simulink model "chap3_2"  (Simulink 5.0)
settings: Solver=ode5  StartTime=0.0  StopTime=500*T  FixedStep=T  RelTol=1e-3
PreLoadFcn:
  | T=0.001; Kp=0.6; Ki=0.03; Kd=0.01;

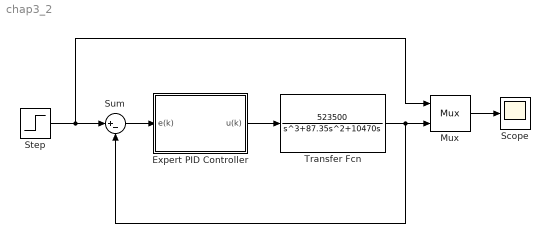
== system chap3_2 ==
  Expert PID Controller : Subsystem  mask{kp=Kp, ki=Ki, kd=Kd, T=0.001, MTab=[0.8,0.45; 0.4,0.4; 0.2,0.12; 0.01 0.1], U_m=10}
      mask prompts: kp "Proportional Kp"; ki "Integral Ki"; kd "Derivative Kd"; T "Sampling period T"; MTab "Mapping Table"; U_m "Actuator Limit U_m"
      mask Display: disp('Expert PID\n Controller')
  Mux : Mux  Inputs=2
  Scope : Scope
      settings: TimeRange=0.5  YMin=-0.0669643  YMax=1.10225  SaveName=yy  DataFormat=Array
  Step : Step  Time=0  SampleTime=0
  Sum : Sum  Inputs=|+-  SaturateOnIntegerOverflow=on  InputSameDT=on
  Transfer Fcn : TransferFcn  Numerator=[523500]  Denominator=[1 87.35 10470 0]
  wires:
  Transfer Fcn/1 -> Sum/2, Mux/2
  Step/1 -> Sum/1, Mux/1
  Expert PID Controller/1(u(k)) -> Transfer Fcn/1
  Sum/1 -> Expert PID Controller/1(e(k))
  Mux/1 -> Scope/1

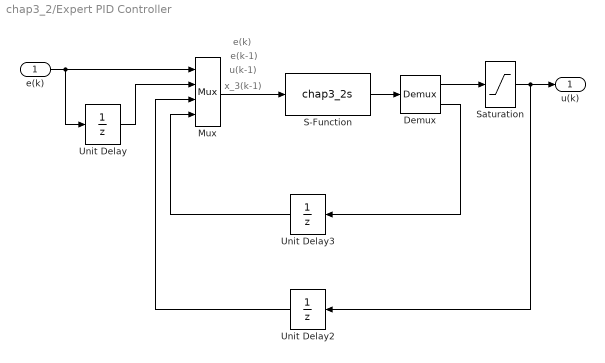
== system chap3_2/Expert PID Controller ==
  note: e(k)
  note: e(k-1)
  note: u(k-1)
  note: x_3(k-1)
  e(k) : Inport
  Demux : Demux  Outputs=2
  Mux : Mux
  S-Function : S-Function  FunctionName=chap3_2s  Parameters=T,Kp,Ki,Kd,MTab
  Saturation : Saturate  UpperLimit=U_m  LowerLimit=-U_m
  Unit Delay : UnitDelay  SampleTime=-1
  Unit Delay2 : UnitDelay  Orientation=left  SampleTime=-1
  Unit Delay3 : UnitDelay  Orientation=left  SampleTime=-1
  u(k) : Outport
  wires:
  Unit Delay2/1 -> Mux/3
  Unit Delay3/1 -> Mux/4
  Demux/2 -> Unit Delay3/1
  e(k)/1 -> Unit Delay/1, Mux/1
  Mux/1 -> S-Function/1
  Unit Delay/1 -> Mux/2
  S-Function/1 -> Demux/1
  Demux/1 -> Saturation/1
  Saturation/1 -> Unit Delay2/1, u(k)/1
